simulink model "myPIDdiscrete"  (R2017a)
settings: Solver=VariableStepAuto  StartTime=0.0  StopTime=50.0  RelTol=1e-3
values from neighbouring files (symbols this model uses):
  A = [(-1/(A1*rh1)),0,0;(1/(A2*rh1)),(-1/(A2*rh2)),0;0,(1/(A3*rh2)),(-1/(A3*rh3))]    [parameters.m]
  B = [1/A1,0,0;0,1/A2,0;0,0,0]    [parameters.m]
  C = [1,0,0;0,1,0;0,0,1]    [parameters.m]
  D = [0,0,0;0,0,0;0,0,0]    [parameters.m]
  kc = 2    [parameters.m]
  T = 1    [parameters.m]
  taud = 0    [parameters.m]
  taui = 5    [parameters.m]
settings Model: Creator=Erebus  LastModifiedBy=Erebus

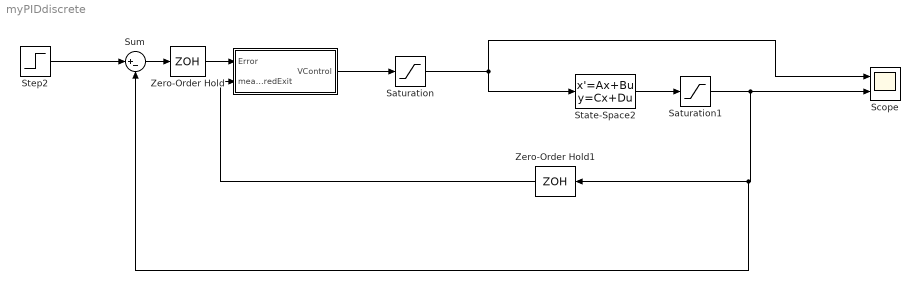
== system myPIDdiscrete ==
  " " : Subsystem
  Saturation : Saturate  UpperLimit=9  LowerLimit=0
  Saturation1 : Saturate  UpperLimit=9  LowerLimit=0
  Scope : Scope  NumInputPorts=2
  State-Space2 : StateSpace  A=A  B=B  C=C  D=D  X0=0
  Step2 : Step  After=[5,7,0]  SampleTime=0
  Sum : Sum  Inputs=|+-
  Zero-Order Hold : ZeroOrderHold  SampleTime=-1
  Zero-Order Hold1 : ZeroOrderHold  SampleTime=-1
  wires:
  Step2/1 -> Sum/1
  Sum/1 -> Zero-Order Hold/1
  Zero-Order Hold/1 -> " "/1(Error)
  Zero-Order Hold1/1 -> " "/2(measuredExit)
  " "/1(VControl) -> Saturation/1
  Saturation/1 -> Scope/1, State-Space2/1
  State-Space2/1 -> Saturation1/1
  Saturation1/1 -> Sum/2, Zero-Order Hold1/1, Scope/2

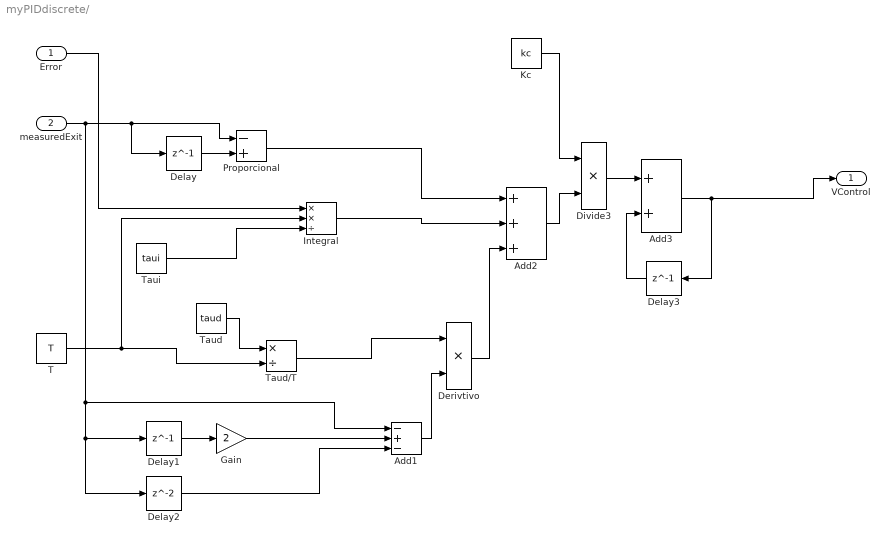
== system myPIDdiscrete/  ==
  Error : Inport
  measuredExit : Inport  Port=2
  Add1 : Sum  Inputs=-+-
  Add2 : Sum  Inputs=+++
  Add3 : Sum
  Delay : Delay  DelayLength=1  SampleTime=T
  Delay1 : Delay  DelayLength=1  SampleTime=T
  Delay2 : Delay  SampleTime=T
  Delay3 : Delay  DelayLength=1  SampleTime=T
  Derivtivo : Product  Inputs=**
  Divide3 : Product  Inputs=**
  Gain : Gain  Gain=2
  Integral : Product  Inputs=**/
  Kc : Constant  Value=kc
  Proporcional : Sum  Inputs=-+
  T : Constant  Value=T
  Taud : Constant  Value=taud
  Taud/T : Product  Inputs=*/
  Taui : Constant  Value=taui
  VControl : Outport
  wires:
  Taud/1 -> Taud/T/1
  T/1 -> Integral/2, Taud/T/2
  Gain/1 -> Add1/2
  Delay/1 -> Proporcional/2
  Kc/1 -> Divide3/1
  Divide3/1 -> Add3/1
  Taui/1 -> Integral/3
  Add1/1 -> Derivtivo/2
  Derivtivo/1 -> Add2/3
  Delay2/1 -> Add1/3
  Add2/1 -> Divide3/2
  measuredExit/1 -> Add1/1, Delay2/1, Delay1/1, Delay/1, Proporcional/1
  Taud/T/1 -> Derivtivo/1
  Delay3/1 -> Add3/2
  Delay1/1 -> Gain/1
  Error/1 -> Integral/1
  Add3/1 -> VControl/1, Delay3/1
  Integral/1 -> Add2/2
  Proporcional/1 -> Add2/1
